simulink model "a_star_test"  (R2017b)
settings: Solver=VariableStepAuto  StartTime=0.0  StopTime=10.0  RelTol=1e-3
settings Model: Creator=jorgeluis  LastModifiedBy=jorgeluis

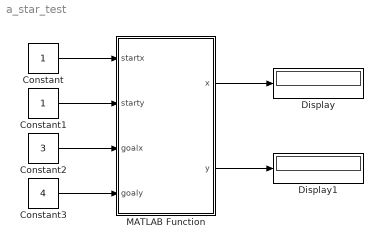
== system a_star_test ==
  Constant : Constant
  Constant1 : Constant
  Constant2 : Constant  Value=3
  Constant3 : Constant  Value=4
  Display : Display
  Display1 : Display
  MATLAB Function : MATLAB Function  TreatAsAtomicUnit=on
  wires:
  MATLAB Function/1(x) -> Display/1
  MATLAB Function/2(y) -> Display1/1
  Constant/1 -> MATLAB Function/1(startx)
  Constant1/1 -> MATLAB Function/2(starty)
  Constant2/1 -> MATLAB Function/3(goalx)
  Constant3/1 -> MATLAB Function/4(goaly)

== matlab function a_star_test/MATLAB Function ==
  data: x output; startx input; y output; starty input; goalx input; goaly input
% Autores: Jorgeluis Guerra
%          Luis Braga
%          Saulo Alves

% Funcao wrapper que insere o algoritmo do A estrela dentro do modelo do
% robo

function [x, y] = wrapper_a_star(startx, starty, goalx, goaly)

   % Valor 'infinito'
   INF = 100000;
   % Limites do grid de celulas
   GRID_MIN = 1;
   GRID_MAX = 5;

   start_node.x = startx;
   start_node.y = starty;
   start_node.g = INF;
   start_node.f = INF;
   start_node.camefrom = [];

   goal_node.x = goalx;
   goal_node.y = goaly;
   goal_node.g = INF;
   goal_node.f = INF;
   goal_node.camefrom = [];

   path_nodes = a_star(start_node, goal_node);

   x = 3;
   y = 4;
   %x = zeros(1, 20);
   %y = zeros(1, 20);
   j = 1;
   %for i = path_nodes
   %   x = i.x;
   %   y = i.y;
   %   j = j + 1;
   %end
end
